simulink model "INDUCTIVE_WIRELESS_CHARGING_FOR_ELECTRIC_VEHICLES"  (R2022b)
settings: Solver=VariableStepAuto  StartTime=0.0  StopTime=10800  RelTol=1e-3
undefined symbols (not defined in the file): Ion, Lithium
libraries: spsDiodeLib x6, spsIGBTDiodeLib x4, spsSeriesRLCBranchLib x3, spsVoltageMeasurementLib x3, spsBatteryLib x1, spsCurrentMeasurementLib x1, spsLinearTransformerLib x1, spsPWMGeneratorDCDCLib x1, eePowerMeasurement x1, spsThreePhaseVIMeasurementLib x1, spsThreePhaseSourceLib x1, spsUniversalBridgeLib x1
settings Model: SimulationMode=accelerator  Creator=deva_  LastModifiedBy=deva_

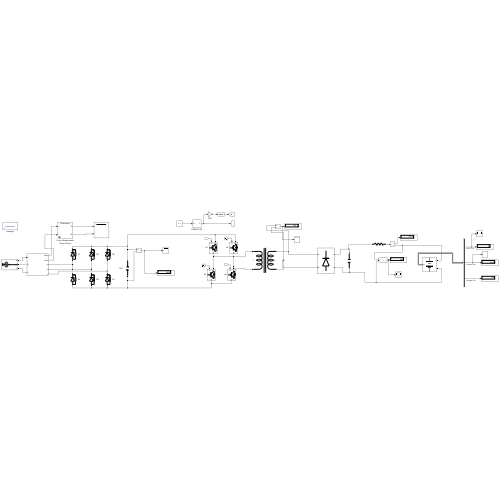
[thumbnail: Simulink's stored preview of the top-level diagram]
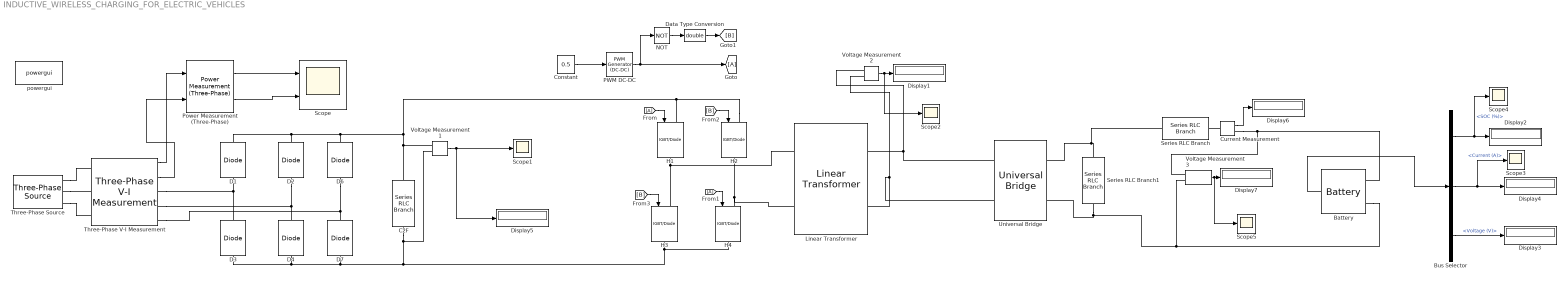
== system INDUCTIVE_WIRELESS_CHARGING_FOR_ELECTRIC_VEHICLES ==
  Battery : spsBatteryLib/Battery  BatType=Lithium-Ion  ShowTempParam=off  ThermalPreset=no  ShowAgeParam=off  NomV=350  NomQ=150  SOC=99  Batt_Tr=30  PresetModel=on  MaxQ=150  MinV=262.5  FullV=407.3955  Dis_rate=65.2174  R=0.023333  Normal_OP=135.6522  expZone="[378.135      7.369565]"  current=[6.5 13 32.5]  Units=Time  Tci=20  NomT=20  T2=-30  MaxQ2=4.8  FullV2=7.1  Normal_OP2=5.655  expZone2="[6.58           1]"  Rca=0.6  ti=2000  Dp=0  Neq0=0  Tsim=1e6  Ta1=25  Qeol=5.4*0.9  Reol=0.013333*1.2  Char_age=[2.3478, 3]  Dis_age=[2.3478, 10]  N1=1500  N2=10500  N3=1000  N4=1400  Ta2=45  N5=950
  Bus Selector : BusSelector  OutputSignals=SOC (%),Current (A),Voltage (V)
  C2F : spsSeriesRLCBranchLib/Series RLC Branch  LConnTagsString=__new0  RConnTagsString=__new0  BranchType=C  Resistance=1e-6  Inductance=1e-3  SetiL0=off  InitialCurrent=0  Capacitance=0.0047  Setx0=off  InitialVoltage=0  Measurements=Branch voltage
  Constant : Constant  Value=0.5
  Current Measurement : spsCurrentMeasurementLib/Current Measurement  PhasorSimulation=off  OutputType=Complex  PSBequivalent=0
  D{1..4,6..7} (6 alike) : spsDiodeLib/Diode  Ron=0.001  Lon=0  Vf=0.7  IC=0  UseSnubber=0  Rs=100000  Cs=Inf  Measurements=off
  Data Type Conversion : DataTypeConversion  OutDataTypeStr=double  SaturateOnIntegerOverflow=off  RndMeth=Floor
  Display{1..7} (7 alike) : Display
  From : From
  From1 : From
  Goto : Goto
  H{1..4} (4 alike) : spsIGBTDiodeLib/IGBT//Diode  Ron=1e-3  Rs=1e5  Cs=inf  Measurements=off
  Linear Transformer : spsLinearTransformerLib/Linear Transformer  UNITS=pu  NominalPower=[12600 30000]  winding1=[540 0.01 0.05]  winding2=[550 0.01 0.05]  ThreeWindings=off  winding3=[3.15e+05 0.002 0.080001]  RmLm=[500 499.99]  Measurements=None  DataType=off
  "NOT " : Logic  Operator=NOT  IconShape=distinctive  AllPortsSameDT=off  OutDataTypeStr=boolean
  PWM DC-DC : spsPWMGeneratorDCDCLib/PWM Generator (DC-DC)  Fsw=30000  Ts=1e-6
  Power Measurement (Three-Phase) : eePowerMeasurement/Power Measurement (Three-Phase)  LabelModeActiveChoice=Continuous  F=60  K=[0 1 2 3]  Seq=Positive  Ts=0
  Scope : Scope  NumInputPorts=2
  Scope{1..5} (5 alike) : Scope
  Series RLC Branch : spsSeriesRLCBranchLib/Series RLC Branch  LConnTagsString=__new0  RConnTagsString=__new0  BranchType=R  Resistance=6.3  Inductance=1e-3  SetiL0=off  InitialCurrent=0  Capacitance=1e-6  Setx0=off  InitialVoltage=0  Measurements=None
  Series RLC Branch1 : spsSeriesRLCBranchLib/Series RLC Branch  LConnTagsString=__new0  RConnTagsString=__new0  BranchType=C  Resistance=1  Inductance=1e-3  SetiL0=off  InitialCurrent=0  Capacitance=0.01  Setx0=off  InitialVoltage=0  Measurements=None
  Three-Phase V-I Measurement : spsThreePhaseVIMeasurementLib/Three-Phase V-I Measurement  VoltageMeasurement=phase-to-ground  SetLabelV=off  LabelV=Vabc  Vpu=off  VpuLL=off  CurrentMeasurement=yes  SetLabelI=off  LabelI=Iabc  Ipu=off  Pbase=100e6  Vbase=500e3  OutputType=Complex  PhasorSimulation=off  PSBequivalent=0
  Three-Phase Source : spsThreePhaseSourceLib/Three-Phase Source  InternalConnection=Yg  VoltagePhases=off  Voltage=430  PhaseAngle=0  Voltage_phases=[25e3 25e3 25e3]/sqrt(3)  PhaseAngles_phases=[0 -120 +120]  Frequency=50  NonIdealSource=off  SpecifyImpedance=off  Resistance=0.8929  Inductance=16.58e-3  ShortCircuitLevel=100e6  BaseVoltage=25e3  XRratio=7  BusType=swing  Pref=10e3  Qref=0  Prefabc=[10e3, 10e3, 10e3]  Qrefabc=[0, 0, 0]  Qmin=-inf  Qmax=inf
  Universal Bridge : spsUniversalBridgeLib/Universal Bridge  Arms=2  SnubberResistance=1e5  SnubberCapacitance=inf  Device=Diodes  Ron=1e-3  Lon=0  ForwardVoltages="[  0  0  ]"  ForwardVoltage=0.7  GTOparameters=[ 10e-6 , 20e-6 ]  IGBTparameters=[ 1e-6 , 2e-6 ]  Measurements=None  Measurements_2=None  converterType=Rectifier
  Voltage Measurement1 : spsVoltageMeasurementLib/Voltage Measurement  PhasorSimulation=off  OutputType=Complex  PSBequivalent=0
  Voltage Measurement2 : spsVoltageMeasurementLib/Voltage Measurement  PhasorSimulation=off  OutputType=Complex  PSBequivalent=0
  Voltage Measurement3 : spsVoltageMeasurementLib/Voltage Measurement  PhasorSimulation=off  OutputType=Complex  PSBequivalent=0
  powergui : spspowerguiLib/powergui  Priority=1  SimulationMode=Continuous  SampleTime=50e-6  frequency=60  Iterations=50  frequencyindice=50  Pbase=100e6  ErrMax=1e-4  UnitsV=kV  UnitsW=MW  buscounter=0  FunctionMessages=off  echomessages=off  EnableUseOfTLC=off  CurrentSourceSwitches=off  DisableSnubberDevices=off  DisableRonSwitches=off  DisableVfSwitches=off  DisplayEquations=off  AutomaticDiscreteSolvers=off  SolverType=Tustin/Backward Euler (TBE)  Interpol=off  ExternalGateDelay=off  methode=off  Ts=100  x0status=blocks  SPID=on  SwTol=0  HookPort=off  NonlinearTolerance=1e-4  nMaxIteration=100  ContinueOnMaxIteration=off  RestoreLinks=warning  ResistiveCurrentMeasurement=off  Frange=[0:2:500]  Ylog=off  Xlog=on  ShowGrid=off  save=off  variable=ZData  structure=0  ZoomFFT=off  StartTime=0.0  cycles=1  DisplayStyle=1  fundamental=60  FreqAxis=off  MaxFrequency=1000  frequencyindicesteady=1  RmsSteady=1  display=off
  wires:
  Voltage Measurement1/1 -> Scope1/1, Display5/1
  Voltage Measurement2/1 -> Scope2/1, Display1/1
  Bus Selector/3 -> Display3/1  "<Voltage (V)>"
  Current Measurement/1 -> Display6/1
  Voltage Measurement3/1 -> Scope5/1, Display7/1
  Battery/1 -> Bus Selector/1
  Bus Selector/2 -> Scope3/1, Display4/1  "<Current (A)>"
  Bus Selector/1 -> Scope4/1, Display2/1  "<SOC (%)>"
  PWM DC-DC/1 -> "NOT "/1, Goto/1
  From/1 -> H1/1
  Data Type Conversion/1 -> [B]
  Constant/1 -> PWM DC-DC/1
  From1/1 -> H4/1
  "NOT "/1 -> Data Type Conversion/1
  [B] -> H3/1
  [B] -> H2/1
  Three-Phase V-I Measurement/1 -> Power Measurement (Three-Phase)/1
  Three-Phase V-I Measurement/2 -> Power Measurement (Three-Phase)/2
  Power Measurement (Three-Phase)/1 -> Scope/1
  Power Measurement (Three-Phase)/2 -> Scope/2
  connections:
  H2/LConn1 -- C2F/LConn1 -- Voltage Measurement1/LConn1 -- D2/RConn1 -- D1/RConn1 -- D6/RConn1 -- H1/LConn1
  H4/RConn1 -- C2F/RConn1 -- Voltage Measurement1/LConn2 -- D7/LConn1 -- D3/LConn1 -- D4/LConn1 -- H3/RConn1
  D2/LConn1 -- Three-Phase V-I Measurement/RConn2 -- D4/RConn1
  D3/RConn1 -- Three-Phase V-I Measurement/RConn1 -- D1/LConn1
  D6/LConn1 -- Three-Phase V-I Measurement/RConn3 -- D7/RConn1
  Voltage Measurement2/LConn2 -- Universal Bridge/LConn2 -- Linear Transformer/RConn2
  Voltage Measurement2/LConn1 -- Universal Bridge/LConn1 -- Linear Transformer/RConn1
  Battery/LConn1 -- Current Measurement/RConn1 -- Voltage Measurement3/LConn1
  Battery/LConn2 -- Series RLC Branch1/RConn1 -- Universal Bridge/RConn2 -- Voltage Measurement3/LConn2
  Universal Bridge/RConn1 -- Series RLC Branch1/LConn1 -- Series RLC Branch/LConn1
  Current Measurement/LConn1 -- Series RLC Branch/RConn1
  H2/RConn1 -- Linear Transformer/LConn2 -- H4/LConn1
  H3/LConn1 -- Linear Transformer/LConn1 -- H1/RConn1
  Three-Phase Source/RConn2 -- Three-Phase V-I Measurement/LConn2
  Three-Phase Source/RConn3 -- Three-Phase V-I Measurement/LConn3
  Three-Phase Source/RConn1 -- Three-Phase V-I Measurement/LConn1
